simulink model "Red_problema7_lazo_abierto_v2021"  (R2021a)
settings: Solver=ode15s  StartTime=0.0  StopTime=sim_time  RelTol=1e-3
values from neighbouring files (symbols this model uses):
  aE1 = a121_f    (= 50.6984417257)    [inicializar_areas_ej7.m]
  aE2 = a112_f    (= 77.7288481128)    [inicializar_areas_ej7.m]
  aE3 = a222_f    (= 163.424628674)    [inicializar_areas_ej7.m]
  aE4 = a213_f    (= 304.960661681)    [inicializar_areas_ej7.m]
  aEcu1 = aEcu1_f    (= 4.92677788377)    [inicializar_areas_ej7.m]
  aEcu2 = aEcu2_f    (= 18.7854640224)    [inicializar_areas_ej7.m]
  aEhu2 = aEhu2_f    (= 81.1441370104)    [inicializar_areas_ej7.m]
  d1_end = 0    [script_build_tfs.m]    (also in todo_nom_full.m; todo_nom_spar.m)
  d1_in = 0    [script_build_tfs.m]    (also in todo_nom_full.m; todo_nom_spar.m)
  d2_end = 0    [script_build_tfs.m]    (also in todo_nom_full.m; todo_nom_spar.m)
  d2_in = 0    [script_build_tfs.m]    (also in todo_nom_full.m; todo_nom_spar.m)
  d3_end = 0    [script_build_tfs.m]    (also in todo_nom_full.m; todo_nom_spar.m)
  d3_in = 0    [script_build_tfs.m]    (also in todo_nom_full.m; todo_nom_spar.m)
  d4_end = 0    [script_build_tfs.m]    (also in todo_nom_full.m; todo_nom_spar.m)
  d4_in = 0    [script_build_tfs.m]    (also in todo_nom_full.m; todo_nom_spar.m)
  d5_end = 0    [script_build_tfs.m]    (also in todo_nom_full.m; todo_nom_spar.m)
  d5_in = 0    [script_build_tfs.m]    (also in todo_nom_full.m; todo_nom_spar.m)
  d6_end = 0    [script_build_tfs.m]    (also in todo_nom_full.m; todo_nom_spar.m)
  d6_in = 0    [script_build_tfs.m]    (also in todo_nom_full.m; todo_nom_spar.m)
  d7_end = 0    [script_build_tfs.m]    (also in todo_nom_full.m; todo_nom_spar.m)
  d7_in = 0    [script_build_tfs.m]    (also in todo_nom_full.m; todo_nom_spar.m)
  d8_end = 0    [script_build_tfs.m]    (also in todo_nom_full.m; todo_nom_spar.m)
  d8_in = 0    [script_build_tfs.m]    (also in todo_nom_full.m; todo_nom_spar.m)
  fcu2 = 5    [ini_comun.m]    (also in inicializar_areas_ej7.m; script_build_tfs.m; script_ini_ej7.m)
  fhu2 = 15    [ini_comun.m]    (also in inicializar_areas_ej7.m; script_build_tfs.m; script_ini_ej7.m)
  hcu = 1    [ini_comun.m]    (also in script_build_tfs.m; script_ini_ej7.m)
  hhu = 1    [ini_comun.m]    (also in script_build_tfs.m; script_ini_ej7.m)
  s1 = 30    [ini_comun.m]    (also in script_build_tfs.m; script_ini_ej7.m)
  salida_pto_op = [432.98548652 333.041991092 482.910853128 483.037830645]    [D_desc_v1.mat]    (also in D_full_v1.mat = [432.959604691 333.033592475 482.878829311 483.126301479]; D_spar_v1.mat = [433.148784168 333.052277913 483.093095371 482.96198908]; salida_pt_op_desc.mat = [432.94450339 332.966292174 482.988443985 483.057252903]; salida_pt_op_desc_v2021.mat)
  t_step = 2000    [ini_comun.m]    (also in script_build_tfs.m = 300; script_ini_ej7.m = 600; validacion.m = 500)
  Tcuin = 288    [ini_comun.m]    (also in script_build_tfs.m; script_ini_ej7.m)
  Thuin = 523    [ini_comun.m]    (also in script_build_tfs.m; script_ini_ej7.m)
  u10_end = nom_ini(10)    [script_build_tfs.m]    (also in todo_nom_full.m = 0; todo_nom_spar.m = 0; validacion.m)
  u10_in = nom_ini(10)    [script_build_tfs.m]    (also in todo_nom_full.m = 0; todo_nom_spar.m = 0; validacion.m)
  u11_end = nom_ini(11)    [script_build_tfs.m]    (also in todo_nom_full.m = 0; todo_nom_spar.m = 0; validacion.m)
  u11_in = nom_ini(11)    [script_build_tfs.m]    (also in todo_nom_full.m = 0; todo_nom_spar.m = 0; validacion.m)
  u1_end = nom_ini(1)    [script_build_tfs.m]    (also in todo_nom_full.m = nominales_u_full(1); todo_nom_spar.m = nominales_u_spar(1); validacion.m)
  u1_in = nom_ini(1)    [script_build_tfs.m]    (also in todo_nom_full.m = nominales_u_full(1); todo_nom_spar.m = nominales_u_spar(1); validacion.m)
  u2_end = nom_ini(2)    [script_build_tfs.m]    (also in todo_nom_full.m = nominales_u_full(2); todo_nom_spar.m = nominales_u_spar(2); validacion.m)
  u2_in = nom_ini(2)    [script_build_tfs.m]    (also in todo_nom_full.m = nominales_u_full(2); todo_nom_spar.m = nominales_u_spar(2); validacion.m)
  u3_end = nom_ini(3)    [script_build_tfs.m]    (also in todo_nom_full.m = nominales_u_full(3); todo_nom_spar.m = nominales_u_spar(3); validacion.m)
  u3_in = nom_ini(3)    [script_build_tfs.m]    (also in todo_nom_full.m = nominales_u_full(3); todo_nom_spar.m = nominales_u_spar(3); validacion.m)
  u4_end = nom_ini(4)    [script_build_tfs.m]    (also in todo_nom_full.m = nominales_u_full(4); todo_nom_spar.m = nominales_u_spar(4); validacion.m)
  u4_in = nom_ini(4)    [script_build_tfs.m]    (also in todo_nom_full.m = nominales_u_full(4); todo_nom_spar.m = nominales_u_spar(4); validacion.m)
  u5_end = nom_ini(5)    [script_build_tfs.m]    (also in todo_nom_full.m = nominales_u_full(5); todo_nom_spar.m = nominales_u_spar(5); validacion.m)
  u5_in = nom_ini(5)    [script_build_tfs.m]    (also in todo_nom_full.m = nominales_u_full(5); todo_nom_spar.m = nominales_u_spar(5); validacion.m)
  u6_end = nom_ini(6)    [script_build_tfs.m]    (also in todo_nom_full.m = nominales_u_full(6); todo_nom_spar.m = nominales_u_spar(6); validacion.m)
  u6_in = nom_ini(6)    [script_build_tfs.m]    (also in todo_nom_full.m = nominales_u_full(6); todo_nom_spar.m = nominales_u_spar(6); validacion.m)
  u7_end = nom_ini(7)    [script_build_tfs.m]    (also in todo_nom_full.m = nominales_u_full(7); todo_nom_spar.m = nominales_u_spar(7); validacion.m)
  u7_in = nom_ini(7)    [script_build_tfs.m]    (also in todo_nom_full.m = nominales_u_full(7); todo_nom_spar.m = nominales_u_spar(7); validacion.m)
  u8_end = nom_ini(8)    [script_build_tfs.m]    (also in todo_nom_full.m = nominales_u_full(8); todo_nom_spar.m = nominales_u_spar(8); validacion.m)
  u8_in = nom_ini(8)    [script_build_tfs.m]    (also in todo_nom_full.m = nominales_u_full(8); todo_nom_spar.m = nominales_u_spar(8); validacion.m)
  u9_end = nom_ini(9)    [script_build_tfs.m]    (also in todo_nom_full.m = 0; todo_nom_spar.m = 0; validacion.m)
  u9_in = nom_ini(9)    [script_build_tfs.m]    (also in todo_nom_full.m = 0; todo_nom_spar.m = 0; validacion.m)
libraries: simulink x5, cstblocks x1
(part 2 of 2)

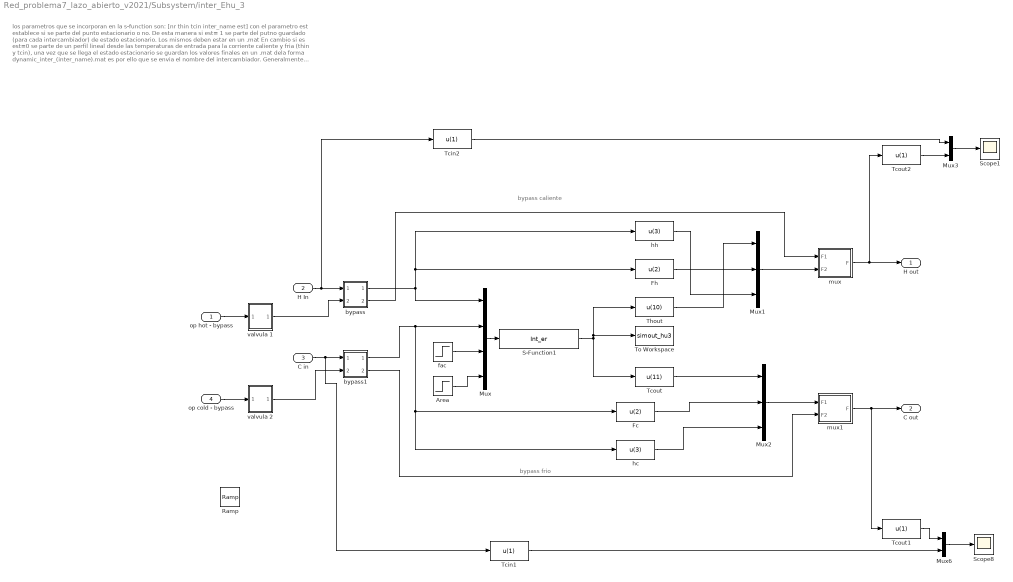
== system Red_problema7_lazo_abierto_v2021/Subsystem/inter_Ehu_3 ==
  note: bypass caliente
  note: bypass frio
  note: los parametros que se incorporan en la s-function son: [nr thin tcin inter_name est]
      | con el parametro est establece si se parte del punto estacionario o no. De esta manera si est= 1 se parte del putno guardado (para cada intercambiador) de estado estacionario. Los mismos deben estar en un .mat
      | En cambio si es est=0 se parte de un perfil lineal  desde las temperaturas de entrada para la corriente caliente y fria (thin y tcin), una vez que se llega el estado estacionario se guardan los valores finales en un .mat
      | dela forma dynamic_inter_(inter_name).mat   es por ello que se envia el nombre del intercambiador.
      | Generalmente para la primera vez que se corre la red se una est=0 para que llegue al estado estacionario y una vez que se alcanzó se vuelve a correr con est= 1 para hacer análisis de control
  "op hot - bypass " : Inport
  H In : Inport  Port=2
  C in : Inport  Port=3
  "op cold - bypass " : Inport  Port=4
  Area : Step  Time=8  Before=aEhu2  After=aEhu2  SampleTime=0
  Fc : Fcn  Expr=u(2)
  Fh : Fcn  Expr=u(2)
  Mux : Mux
  Mux1 : Mux  Inputs=3
  Mux2 : Mux  Inputs=3
  Mux3 : Mux  Inputs=2
  Mux6 : Mux  Inputs=2
  Ramp : simulink/Sources/Ramp  slope=1  start=0  InitialOutput=0
  S-Function1 : S-Function  FunctionName=Int_er  Parameters=10 523 471 03 2  SFunctionDeploymentMode=off  EnableBusSupport=off
  Scope1 : Scope
  Scope8 : Scope
  Tcin1 : Fcn  Expr=u(1)
  Tcin2 : Fcn  Expr=u(1)
  Tcout : Fcn  Expr=u(11)
  Tcout1 : Fcn  Expr=u(1)
  Tcout2 : Fcn  Expr=u(1)
  Thout : Fcn  Expr=u(10)
  To Workspace : ToWorkspace  VariableName=simout_hu3  SampleTime=-1
  bypass : Subsystem
  bypass1 : Subsystem
  fac : Step  After=0  SampleTime=0
  hc : Fcn  Expr=u(3)
  hh : Fcn  Expr=u(3)
  mux : Subsystem
  mux1 : Subsystem
  valvula 1 : Subsystem
  valvula 2 : Subsystem
  H out : Outport  VectorParamsAs1DForOutWhenUnconnected=off
  C out : Outport  Port=2  VectorParamsAs1DForOutWhenUnconnected=off
  wires:
  Tcin2/1 -> Mux3/1
  Tcout2/1 -> Mux3/2
  Mux3/1 -> Scope1/1
  Tcin1/1 -> Mux6/2
  Tcout1/1 -> Mux6/1
  Mux6/1 -> Scope8/1
  bypass1/2(" 2") -> mux1/2(F2)
  bypass1/1(" 1") -> Mux/2, Fc/1, hc/1
  mux1/1("F ") -> C out/1, Tcout1/1
  Mux2/1 -> mux1/1(F1)
  mux/1("F ") -> H out/1, Tcout2/1
  "op cold - bypass "/1 -> valvula 2/1(In1)
  C in/1 -> bypass1/1(1), Tcin1/1
  "op hot - bypass "/1 -> valvula 1/1(In1)
  bypass/2(" 2") -> mux/1(F1)
  Mux1/1 -> mux/2(F2)
  bypass/1(" 1") -> hh/1, Fh/1, Mux/1
  H In/1 -> bypass/1(1), Tcin2/1
  Area/1 -> Mux/4
  hh/1 -> Mux1/3
  hc/1 -> Mux2/3
  fac/1 -> Mux/3
  Mux/1 -> S-Function1/1
  S-Function1/1 -> Tcout/1, To Workspace/1, Thout/1
  Fh/1 -> Mux1/2
  Fc/1 -> Mux2/2
  Thout/1 -> Mux1/1
  Tcout/1 -> Mux2/1
  valvula 1/1(Out1) -> bypass/2(u122)
  valvula 2/1(Out1) -> bypass1/2(u122)

== system Red_problema7_lazo_abierto_v2021/Subsystem/Corriente C1/valvula 3 ==
  In1 : Inport
  Gain : Gain  Gain=s1
  Gain1 : Gain  Gain=s1
  Integrator : Integrator  InitialCondition=[Thuin fhu2 hhu]
  Sum : Sum  Inputs=|+-
  Out1 : Outport  VectorParamsAs1DForOutWhenUnconnected=off
  wires:
  Gain1/1 -> Sum/2
  Integrator/1 -> Out1/1, Gain1/1
  Sum/1 -> Integrator/1
  Gain/1 -> Sum/1
  In1/1 -> Gain/1

== system Red_problema7_lazo_abierto_v2021/Subsystem/Corriente C2/valvula 3 ==
  In1 : Inport
  Gain : Gain  Gain=s1
  Gain1 : Gain  Gain=s1
  Integrator : Integrator  InitialCondition=[Thuin fhu2 hhu]
  Sum : Sum  Inputs=|+-
  Out1 : Outport  VectorParamsAs1DForOutWhenUnconnected=off
  wires:
  Gain1/1 -> Sum/2
  Integrator/1 -> Out1/1, Gain1/1
  Sum/1 -> Integrator/1
  Gain/1 -> Sum/1
  In1/1 -> Gain/1

== system Red_problema7_lazo_abierto_v2021/Subsystem/Corriente H1/valvula 3 ==
  In1 : Inport
  Gain : Gain  Gain=s1
  Gain1 : Gain  Gain=s1
  Integrator : Integrator  InitialCondition=[Thuin fhu2 hhu]
  Sum : Sum  Inputs=|+-
  Out1 : Outport  VectorParamsAs1DForOutWhenUnconnected=off
  wires:
  Gain1/1 -> Sum/2
  Integrator/1 -> Out1/1, Gain1/1
  Sum/1 -> Integrator/1
  Gain/1 -> Sum/1
  In1/1 -> Gain/1

== system Red_problema7_lazo_abierto_v2021/Subsystem/Corriente H2/valvula 3 ==
  In1 : Inport
  Gain : Gain  Gain=s1
  Gain1 : Gain  Gain=s1
  Integrator : Integrator  InitialCondition=[Thuin fhu2 hhu]
  Sum : Sum  Inputs=|+-
  Out1 : Outport  VectorParamsAs1DForOutWhenUnconnected=off
  wires:
  Gain1/1 -> Sum/2
  Integrator/1 -> Out1/1, Gain1/1
  Sum/1 -> Integrator/1
  Gain/1 -> Sum/1
  In1/1 -> Gain/1

== system Red_problema7_lazo_abierto_v2021/Subsystem/Corriente Hu1/valvula 3 ==
  In1 : Inport
  Gain : Gain  Gain=s1
  Gain1 : Gain  Gain=s1
  Integrator : Integrator  InitialCondition=[Tcuin fcu2 hcu]
  Sum : Sum  Inputs=|+-
  Out1 : Outport  VectorParamsAs1DForOutWhenUnconnected=off
  wires:
  Gain1/1 -> Sum/2
  Integrator/1 -> Out1/1, Gain1/1
  Sum/1 -> Integrator/1
  Gain/1 -> Sum/1
  In1/1 -> Gain/1

== system Red_problema7_lazo_abierto_v2021/Subsystem/Corriente Hu2/valvula 3 ==
  In1 : Inport
  Gain : Gain  Gain=s1
  Gain1 : Gain  Gain=s1
  Integrator : Integrator  InitialCondition=[Tcuin fcu2 hcu]
  Sum : Sum  Inputs=|+-
  Out1 : Outport  VectorParamsAs1DForOutWhenUnconnected=off
  wires:
  Gain1/1 -> Sum/2
  Integrator/1 -> Out1/1, Gain1/1
  Sum/1 -> Integrator/1
  Gain/1 -> Sum/1
  In1/1 -> Gain/1

== system Red_problema7_lazo_abierto_v2021/Subsystem/Corriente Hu3/valvula 3 ==
  In1 : Inport
  Gain : Gain  Gain=s1
  Gain1 : Gain  Gain=s1
  Integrator : Integrator  InitialCondition=[Tcuin fcu2 hcu]
  Sum : Sum  Inputs=|+-
  Out1 : Outport  VectorParamsAs1DForOutWhenUnconnected=off
  wires:
  Gain1/1 -> Sum/2
  Integrator/1 -> Out1/1, Gain1/1
  Sum/1 -> Integrator/1
  Gain/1 -> Sum/1
  In1/1 -> Gain/1

== system Red_problema7_lazo_abierto_v2021/Subsystem/inter_E1/bypass ==
  note: la corriete 2 es la corriente del byapass
  note: la corriente 1 es la que se introduce al intercambiador
  1 : Inport
  u122 : Inport  Port=2
  Add : Sum  Inputs=+-
  Mux : Mux  Inputs=3
  Mux1 : Mux  Inputs=3
  Product : Product
  T : Fcn  Expr=u(1)
  f : Fcn  Expr=u(2)
  h : Fcn  Expr=u(3)
  " 1" : Outport  VectorParamsAs1DForOutWhenUnconnected=off
  " 2" : Outport  Port=2  VectorParamsAs1DForOutWhenUnconnected=off
  wires:
  u122/1 -> Product/1
  f/1 -> Add/1, Product/2
  Product/1 -> Mux1/2, Add/2
  1/1 -> T/1, h/1, f/1
  Add/1 -> Mux/2
  h/1 -> Mux1/3, Mux/3
  T/1 -> Mux1/1, Mux/1
  Mux/1 -> " 1"/1
  Mux1/1 -> " 2"/1

== system Red_problema7_lazo_abierto_v2021/Subsystem/inter_E1/bypass1 ==
  note: la corriente 1 es la que se introduce al intercambiador
  note: la corriete 2 es la corriente del byapass
  1 : Inport
  u122 : Inport  Port=2
  Add : Sum  Inputs=+-
  Mux : Mux  Inputs=3
  Mux1 : Mux  Inputs=3
  Product : Product
  T : Fcn  Expr=u(1)
  f : Fcn  Expr=u(2)
  h : Fcn  Expr=u(3)
  " 1" : Outport  VectorParamsAs1DForOutWhenUnconnected=off
  " 2" : Outport  Port=2  VectorParamsAs1DForOutWhenUnconnected=off
  wires:
  Mux1/1 -> " 2"/1
  Mux/1 -> " 1"/1
  T/1 -> Mux/1, Mux1/1
  h/1 -> Mux/3, Mux1/3
  Add/1 -> Mux/2
  1/1 -> f/1, h/1, T/1
  Product/1 -> Add/2, Mux1/2
  f/1 -> Product/2, Add/1
  u122/1 -> Product/1

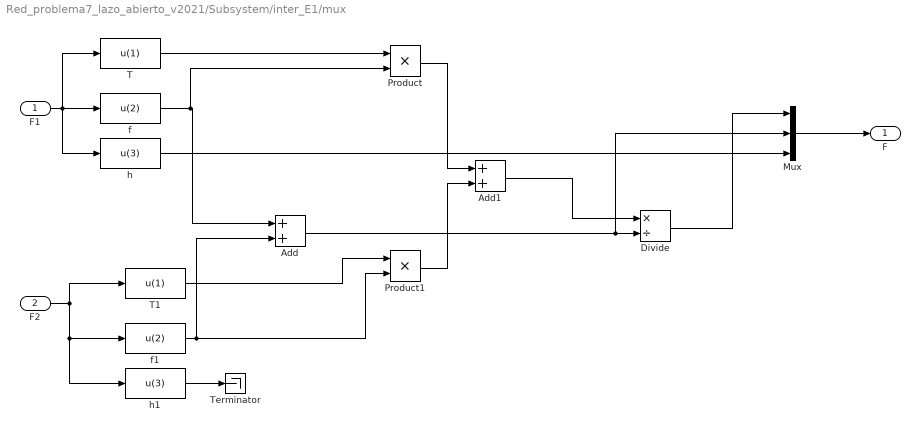
== system Red_problema7_lazo_abierto_v2021/Subsystem/inter_E1/mux ==
  F1 : Inport
  F2 : Inport  Port=2
  Add : Sum
  Add1 : Sum
  Divide : Product  Inputs=*/
  Mux : Mux  Inputs=3
  Product : Product
  Product1 : Product
  T : Fcn  Expr=u(1)
  T1 : Fcn  Expr=u(1)
  Terminator : Terminator
  f : Fcn  Expr=u(2)
  f1 : Fcn  Expr=u(2)
  h : Fcn  Expr=u(3)
  h1 : Fcn  Expr=u(3)
  "F " : Outport  VectorParamsAs1DForOutWhenUnconnected=off
  wires:
  h/1 -> Mux/3
  Divide/1 -> Mux/1
  Add/1 -> Divide/2, Mux/2
  Add1/1 -> Divide/1
  Product1/1 -> Add1/2
  f1/1 -> Product1/2, Add/2
  T1/1 -> Product1/1
  Product/1 -> Add1/1
  T/1 -> Product/1
  F2/1 -> T1/1, f1/1, h1/1
  f/1 -> Add/1, Product/2
  F1/1 -> T/1, h/1, f/1
  Mux/1 -> "F "/1
  h1/1 -> Terminator/1

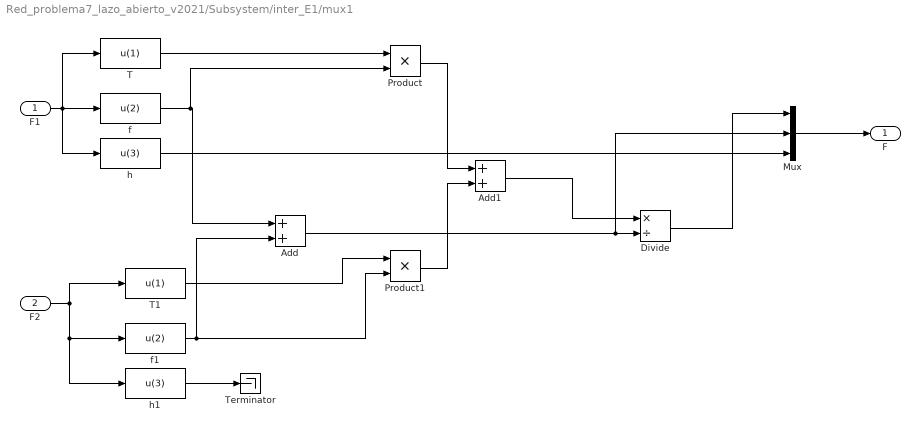
== system Red_problema7_lazo_abierto_v2021/Subsystem/inter_E1/mux1 ==
  F1 : Inport
  F2 : Inport  Port=2
  Add : Sum
  Add1 : Sum
  Divide : Product  Inputs=*/
  Mux : Mux  Inputs=3
  Product : Product
  Product1 : Product
  T : Fcn  Expr=u(1)
  T1 : Fcn  Expr=u(1)
  Terminator : Terminator
  f : Fcn  Expr=u(2)
  f1 : Fcn  Expr=u(2)
  h : Fcn  Expr=u(3)
  h1 : Fcn  Expr=u(3)
  "F " : Outport  VectorParamsAs1DForOutWhenUnconnected=off
  wires:
  Mux/1 -> "F "/1
  F1/1 -> f/1, h/1, T/1
  f/1 -> Product/2, Add/1
  F2/1 -> h1/1, f1/1, T1/1
  T/1 -> Product/1
  Product/1 -> Add1/1
  T1/1 -> Product1/1
  f1/1 -> Add/2, Product1/2
  Product1/1 -> Add1/2
  Add1/1 -> Divide/1
  Add/1 -> Mux/2, Divide/2
  Divide/1 -> Mux/1
  h/1 -> Mux/3
  h1/1 -> Terminator/1

== system Red_problema7_lazo_abierto_v2021/Subsystem/inter_E1/valvula 1 ==
  In1 : Inport
  Gain : Gain  Gain=s1
  Gain1 : Gain  Gain=s1
  Integrator : Integrator
  Sum : Sum  Inputs=|+-
  Out1 : Outport  VectorParamsAs1DForOutWhenUnconnected=off
  wires:
  Gain1/1 -> Sum/2
  Integrator/1 -> Out1/1, Gain1/1
  Sum/1 -> Integrator/1
  Gain/1 -> Sum/1
  In1/1 -> Gain/1

== system Red_problema7_lazo_abierto_v2021/Subsystem/inter_E1/valvula 2 ==
  In1 : Inport
  Gain : Gain  Gain=s1
  Gain1 : Gain  Gain=s1
  Integrator : Integrator
  Sum : Sum  Inputs=|+-
  Out1 : Outport  VectorParamsAs1DForOutWhenUnconnected=off
  wires:
  Gain1/1 -> Sum/2
  Integrator/1 -> Out1/1, Gain1/1
  Sum/1 -> Integrator/1
  Gain/1 -> Sum/1
  In1/1 -> Gain/1

== system Red_problema7_lazo_abierto_v2021/Subsystem/inter_E2/bypass ==
  note: la corriente 1 es la que se introduce al intercambiador
  note: la corriete 2 es la corriente del byapass
  1 : Inport
  u122 : Inport  Port=2
  Add : Sum  Inputs=+-
  Mux : Mux  Inputs=3
  Mux1 : Mux  Inputs=3
  Product : Product
  T : Fcn  Expr=u(1)
  f : Fcn  Expr=u(2)
  h : Fcn  Expr=u(3)
  " 1" : Outport  VectorParamsAs1DForOutWhenUnconnected=off
  " 2" : Outport  Port=2  VectorParamsAs1DForOutWhenUnconnected=off
  wires:
  Mux1/1 -> " 2"/1
  Mux/1 -> " 1"/1
  T/1 -> Mux/1, Mux1/1
  h/1 -> Mux/3, Mux1/3
  Add/1 -> Mux/2
  1/1 -> f/1, h/1, T/1
  Product/1 -> Add/2, Mux1/2
  f/1 -> Product/2, Add/1
  u122/1 -> Product/1

== system Red_problema7_lazo_abierto_v2021/Subsystem/inter_E2/bypass1 ==
  note: la corriete 2 es la corriente del byapass
  note: la corriente 1 es la que se introduce al intercambiador
  1 : Inport
  u122 : Inport  Port=2
  Add : Sum  Inputs=+-
  Mux : Mux  Inputs=3
  Mux1 : Mux  Inputs=3
  Product : Product
  T : Fcn  Expr=u(1)
  f : Fcn  Expr=u(2)
  h : Fcn  Expr=u(3)
  " 1" : Outport  VectorParamsAs1DForOutWhenUnconnected=off
  " 2" : Outport  Port=2  VectorParamsAs1DForOutWhenUnconnected=off
  wires:
  u122/1 -> Product/1
  f/1 -> Add/1, Product/2
  Product/1 -> Mux1/2, Add/2
  1/1 -> T/1, h/1, f/1
  Add/1 -> Mux/2
  h/1 -> Mux1/3, Mux/3
  T/1 -> Mux1/1, Mux/1
  Mux/1 -> " 1"/1
  Mux1/1 -> " 2"/1

== system Red_problema7_lazo_abierto_v2021/Subsystem/inter_E2/mux ==
  F1 : Inport
  F2 : Inport  Port=2
  Add : Sum
  Add1 : Sum
  Divide : Product  Inputs=*/
  Mux : Mux  Inputs=3
  Product : Product
  Product1 : Product
  T : Fcn  Expr=u(1)
  T1 : Fcn  Expr=u(1)
  f : Fcn  Expr=u(2)
  f1 : Fcn  Expr=u(2)
  h : Fcn  Expr=u(3)
  h1 : Fcn  Expr=u(3)
  "F " : Outport  VectorParamsAs1DForOutWhenUnconnected=off
  wires:
  Mux/1 -> "F "/1
  F1/1 -> f/1, h/1, T/1
  f/1 -> Product/2, Add/1
  F2/1 -> h1/1, f1/1, T1/1
  T/1 -> Product/1
  Product/1 -> Add1/1
  T1/1 -> Product1/1
  f1/1 -> Add/2, Product1/2
  Product1/1 -> Add1/2
  Add1/1 -> Divide/1
  Add/1 -> Mux/2, Divide/2
  Divide/1 -> Mux/1
  h/1 -> Mux/3

== system Red_problema7_lazo_abierto_v2021/Subsystem/inter_E2/mux1 ==
  F1 : Inport
  F2 : Inport  Port=2
  Add : Sum
  Add1 : Sum
  Divide : Product  Inputs=*/
  Mux : Mux  Inputs=3
  Product : Product
  Product1 : Product
  T : Fcn  Expr=u(1)
  T1 : Fcn  Expr=u(1)
  f : Fcn  Expr=u(2)
  f1 : Fcn  Expr=u(2)
  h : Fcn  Expr=u(3)
  h1 : Fcn  Expr=u(3)
  "F " : Outport  VectorParamsAs1DForOutWhenUnconnected=off
  wires:
  h/1 -> Mux/3
  Divide/1 -> Mux/1
  Add/1 -> Divide/2, Mux/2
  Add1/1 -> Divide/1
  Product1/1 -> Add1/2
  f1/1 -> Product1/2, Add/2
  T1/1 -> Product1/1
  Product/1 -> Add1/1
  T/1 -> Product/1
  F2/1 -> T1/1, f1/1, h1/1
  f/1 -> Add/1, Product/2
  F1/1 -> T/1, h/1, f/1
  Mux/1 -> "F "/1

== system Red_problema7_lazo_abierto_v2021/Subsystem/inter_E2/valvula 1 ==
  In1 : Inport
  Gain : Gain  Gain=s1
  Gain1 : Gain  Gain=s1
  Integrator : Integrator
  Sum : Sum  Inputs=|+-
  Out1 : Outport  VectorParamsAs1DForOutWhenUnconnected=off
  wires:
  Gain1/1 -> Sum/2
  Integrator/1 -> Out1/1, Gain1/1
  Sum/1 -> Integrator/1
  Gain/1 -> Sum/1
  In1/1 -> Gain/1

== system Red_problema7_lazo_abierto_v2021/Subsystem/inter_E2/valvula 2 ==
  In1 : Inport
  Gain : Gain  Gain=s1
  Gain1 : Gain  Gain=s1
  Integrator : Integrator
  Sum : Sum  Inputs=|+-
  Out1 : Outport  VectorParamsAs1DForOutWhenUnconnected=off
  wires:
  Gain1/1 -> Sum/2
  Integrator/1 -> Out1/1, Gain1/1
  Sum/1 -> Integrator/1
  Gain/1 -> Sum/1
  In1/1 -> Gain/1

== system Red_problema7_lazo_abierto_v2021/Subsystem/inter_E3/bypass ==
  note: la corriente 1 es la que se introduce al intercambiador
  note: la corriete 2 es la corriente del byapass
  1 : Inport
  u122 : Inport  Port=2
  Add : Sum  Inputs=+-
  Mux : Mux  Inputs=3
  Mux1 : Mux  Inputs=3
  Product : Product
  T : Fcn  Expr=u(1)
  f : Fcn  Expr=u(2)
  h : Fcn  Expr=u(3)
  " 1" : Outport  VectorParamsAs1DForOutWhenUnconnected=off
  " 2" : Outport  Port=2  VectorParamsAs1DForOutWhenUnconnected=off
  wires:
  Mux1/1 -> " 2"/1
  Mux/1 -> " 1"/1
  T/1 -> Mux/1, Mux1/1
  h/1 -> Mux/3, Mux1/3
  Add/1 -> Mux/2
  1/1 -> f/1, h/1, T/1
  Product/1 -> Add/2, Mux1/2
  f/1 -> Product/2, Add/1
  u122/1 -> Product/1

== system Red_problema7_lazo_abierto_v2021/Subsystem/inter_E3/bypass1 ==
  note: la corriete 2 es la corriente del byapass
  note: la corriente 1 es la que se introduce al intercambiador
  1 : Inport
  u122 : Inport  Port=2
  Add : Sum  Inputs=+-
  Mux : Mux  Inputs=3
  Mux1 : Mux  Inputs=3
  Product : Product
  T : Fcn  Expr=u(1)
  f : Fcn  Expr=u(2)
  h : Fcn  Expr=u(3)
  " 1" : Outport  VectorParamsAs1DForOutWhenUnconnected=off
  " 2" : Outport  Port=2  VectorParamsAs1DForOutWhenUnconnected=off
  wires:
  u122/1 -> Product/1
  f/1 -> Add/1, Product/2
  Product/1 -> Mux1/2, Add/2
  1/1 -> T/1, h/1, f/1
  Add/1 -> Mux/2
  h/1 -> Mux1/3, Mux/3
  T/1 -> Mux1/1, Mux/1
  Mux/1 -> " 1"/1
  Mux1/1 -> " 2"/1

== system Red_problema7_lazo_abierto_v2021/Subsystem/inter_E3/mux ==
  F1 : Inport
  F2 : Inport  Port=2
  Add : Sum
  Add1 : Sum
  Divide : Product  Inputs=*/
  Mux : Mux  Inputs=3
  Product : Product
  Product1 : Product
  T : Fcn  Expr=u(1)
  T1 : Fcn  Expr=u(1)
  f : Fcn  Expr=u(2)
  f1 : Fcn  Expr=u(2)
  h : Fcn  Expr=u(3)
  h1 : Fcn  Expr=u(3)
  "F " : Outport  VectorParamsAs1DForOutWhenUnconnected=off
  wires:
  Mux/1 -> "F "/1
  F1/1 -> f/1, h/1, T/1
  f/1 -> Product/2, Add/1
  F2/1 -> h1/1, f1/1, T1/1
  T/1 -> Product/1
  Product/1 -> Add1/1
  T1/1 -> Product1/1
  f1/1 -> Add/2, Product1/2
  Product1/1 -> Add1/2
  Add1/1 -> Divide/1
  Add/1 -> Mux/2, Divide/2
  Divide/1 -> Mux/1
  h/1 -> Mux/3

== system Red_problema7_lazo_abierto_v2021/Subsystem/inter_E3/mux1 ==
  F1 : Inport
  F2 : Inport  Port=2
  Add : Sum
  Add1 : Sum
  Divide : Product  Inputs=*/
  Mux : Mux  Inputs=3
  Product : Product
  Product1 : Product
  T : Fcn  Expr=u(1)
  T1 : Fcn  Expr=u(1)
  f : Fcn  Expr=u(2)
  f1 : Fcn  Expr=u(2)
  h : Fcn  Expr=u(3)
  h1 : Fcn  Expr=u(3)
  "F " : Outport  VectorParamsAs1DForOutWhenUnconnected=off
  wires:
  h/1 -> Mux/3
  Divide/1 -> Mux/1
  Add/1 -> Divide/2, Mux/2
  Add1/1 -> Divide/1
  Product1/1 -> Add1/2
  f1/1 -> Product1/2, Add/2
  T1/1 -> Product1/1
  Product/1 -> Add1/1
  T/1 -> Product/1
  F2/1 -> T1/1, f1/1, h1/1
  f/1 -> Add/1, Product/2
  F1/1 -> T/1, h/1, f/1
  Mux/1 -> "F "/1

== system Red_problema7_lazo_abierto_v2021/Subsystem/inter_E3/valvula 1 ==
  In1 : Inport
  Gain : Gain  Gain=s1
  Gain1 : Gain  Gain=s1
  Integrator : Integrator
  Sum : Sum  Inputs=|+-
  Out1 : Outport  VectorParamsAs1DForOutWhenUnconnected=off
  wires:
  Gain1/1 -> Sum/2
  Integrator/1 -> Out1/1, Gain1/1
  Sum/1 -> Integrator/1
  Gain/1 -> Sum/1
  In1/1 -> Gain/1

== system Red_problema7_lazo_abierto_v2021/Subsystem/inter_E3/valvula 2 ==
  In1 : Inport
  Gain : Gain  Gain=s1
  Gain1 : Gain  Gain=s1
  Integrator : Integrator
  Sum : Sum  Inputs=|+-
  Out1 : Outport  VectorParamsAs1DForOutWhenUnconnected=off
  wires:
  Gain1/1 -> Sum/2
  Integrator/1 -> Out1/1, Gain1/1
  Sum/1 -> Integrator/1
  Gain/1 -> Sum/1
  In1/1 -> Gain/1

== system Red_problema7_lazo_abierto_v2021/Subsystem/inter_E4/bypass ==
  note: la corriente 1 es la que se introduce al intercambiador
  note: la corriete 2 es la corriente del byapass
  1 : Inport
  u122 : Inport  Port=2
  Add : Sum  Inputs=+-
  Mux : Mux  Inputs=3
  Mux1 : Mux  Inputs=3
  Product : Product
  T : Fcn  Expr=u(1)
  f : Fcn  Expr=u(2)
  h : Fcn  Expr=u(3)
  " 1" : Outport  VectorParamsAs1DForOutWhenUnconnected=off
  " 2" : Outport  Port=2  VectorParamsAs1DForOutWhenUnconnected=off
  wires:
  Mux1/1 -> " 2"/1
  Mux/1 -> " 1"/1
  T/1 -> Mux/1, Mux1/1
  h/1 -> Mux/3, Mux1/3
  Add/1 -> Mux/2
  1/1 -> f/1, h/1, T/1
  Product/1 -> Add/2, Mux1/2
  f/1 -> Product/2, Add/1
  u122/1 -> Product/1

== system Red_problema7_lazo_abierto_v2021/Subsystem/inter_E4/bypass1 ==
  note: la corriete 2 es la corriente del byapass
  note: la corriente 1 es la que se introduce al intercambiador
  1 : Inport
  u122 : Inport  Port=2
  Add : Sum  Inputs=+-
  Mux : Mux  Inputs=3
  Mux1 : Mux  Inputs=3
  Product : Product
  T : Fcn  Expr=u(1)
  f : Fcn  Expr=u(2)
  h : Fcn  Expr=u(3)
  " 1" : Outport  VectorParamsAs1DForOutWhenUnconnected=off
  " 2" : Outport  Port=2  VectorParamsAs1DForOutWhenUnconnected=off
  wires:
  u122/1 -> Product/1
  f/1 -> Add/1, Product/2
  Product/1 -> Mux1/2, Add/2
  1/1 -> T/1, h/1, f/1
  Add/1 -> Mux/2
  h/1 -> Mux1/3, Mux/3
  T/1 -> Mux1/1, Mux/1
  Mux/1 -> " 1"/1
  Mux1/1 -> " 2"/1

== system Red_problema7_lazo_abierto_v2021/Subsystem/inter_E4/mux ==
  F1 : Inport
  F2 : Inport  Port=2
  Add : Sum
  Add1 : Sum
  Divide : Product  Inputs=*/
  Mux : Mux  Inputs=3
  Product : Product
  Product1 : Product
  T : Fcn  Expr=u(1)
  T1 : Fcn  Expr=u(1)
  f : Fcn  Expr=u(2)
  f1 : Fcn  Expr=u(2)
  h : Fcn  Expr=u(3)
  h1 : Fcn  Expr=u(3)
  "F " : Outport  VectorParamsAs1DForOutWhenUnconnected=off
  wires:
  Mux/1 -> "F "/1
  F1/1 -> f/1, h/1, T/1
  f/1 -> Product/2, Add/1
  F2/1 -> h1/1, f1/1, T1/1
  T/1 -> Product/1
  Product/1 -> Add1/1
  T1/1 -> Product1/1
  f1/1 -> Add/2, Product1/2
  Product1/1 -> Add1/2
  Add1/1 -> Divide/1
  Add/1 -> Mux/2, Divide/2
  Divide/1 -> Mux/1
  h/1 -> Mux/3

== system Red_problema7_lazo_abierto_v2021/Subsystem/inter_E4/mux1 ==
  F1 : Inport
  F2 : Inport  Port=2
  Add : Sum
  Add1 : Sum
  Divide : Product  Inputs=*/
  Mux : Mux  Inputs=3
  Product : Product
  Product1 : Product
  T : Fcn  Expr=u(1)
  T1 : Fcn  Expr=u(1)
  f : Fcn  Expr=u(2)
  f1 : Fcn  Expr=u(2)
  h : Fcn  Expr=u(3)
  h1 : Fcn  Expr=u(3)
  "F " : Outport  VectorParamsAs1DForOutWhenUnconnected=off
  wires:
  h/1 -> Mux/3
  Divide/1 -> Mux/1
  Add/1 -> Divide/2, Mux/2
  Add1/1 -> Divide/1
  Product1/1 -> Add1/2
  f1/1 -> Product1/2, Add/2
  T1/1 -> Product1/1
  Product/1 -> Add1/1
  T/1 -> Product/1
  F2/1 -> T1/1, f1/1, h1/1
  f/1 -> Add/1, Product/2
  F1/1 -> T/1, h/1, f/1
  Mux/1 -> "F "/1

== system Red_problema7_lazo_abierto_v2021/Subsystem/inter_E4/valvula 1 ==
  In1 : Inport
  Gain : Gain  Gain=s1
  Gain1 : Gain  Gain=s1
  Integrator : Integrator
  Sum : Sum  Inputs=|+-
  Out1 : Outport  VectorParamsAs1DForOutWhenUnconnected=off
  wires:
  Gain1/1 -> Sum/2
  Integrator/1 -> Out1/1, Gain1/1
  Sum/1 -> Integrator/1
  Gain/1 -> Sum/1
  In1/1 -> Gain/1

== system Red_problema7_lazo_abierto_v2021/Subsystem/inter_E4/valvula 2 ==
  In1 : Inport
  Gain : Gain  Gain=s1
  Gain1 : Gain  Gain=s1
  Integrator : Integrator
  Sum : Sum  Inputs=|+-
  Out1 : Outport  VectorParamsAs1DForOutWhenUnconnected=off
  wires:
  Gain1/1 -> Sum/2
  Integrator/1 -> Out1/1, Gain1/1
  Sum/1 -> Integrator/1
  Gain/1 -> Sum/1
  In1/1 -> Gain/1

== system Red_problema7_lazo_abierto_v2021/Subsystem/inter_Ecu_1/bypass ==
  note: la corriente 1 es la que se introduce al intercambiador
  note: la corriete 2 es la corriente del byapass
  1 : Inport
  u122 : Inport  Port=2
  Add : Sum  Inputs=+-
  Mux : Mux  Inputs=3
  Mux1 : Mux  Inputs=3
  Product : Product
  T : Fcn  Expr=u(1)
  f : Fcn  Expr=u(2)
  h : Fcn  Expr=u(3)
  " 1" : Outport  VectorParamsAs1DForOutWhenUnconnected=off
  " 2" : Outport  Port=2  VectorParamsAs1DForOutWhenUnconnected=off
  wires:
  Mux1/1 -> " 2"/1
  Mux/1 -> " 1"/1
  T/1 -> Mux/1, Mux1/1
  h/1 -> Mux/3, Mux1/3
  Add/1 -> Mux/2
  1/1 -> f/1, h/1, T/1
  Product/1 -> Add/2, Mux1/2
  f/1 -> Product/2, Add/1
  u122/1 -> Product/1

== system Red_problema7_lazo_abierto_v2021/Subsystem/inter_Ecu_1/bypass1 ==
  note: la corriete 2 es la corriente del byapass
  note: la corriente 1 es la que se introduce al intercambiador
  1 : Inport
  u122 : Inport  Port=2
  Add : Sum  Inputs=+-
  Mux : Mux  Inputs=3
  Mux1 : Mux  Inputs=3
  Product : Product
  T : Fcn  Expr=u(1)
  f : Fcn  Expr=u(2)
  h : Fcn  Expr=u(3)
  " 1" : Outport  VectorParamsAs1DForOutWhenUnconnected=off
  " 2" : Outport  Port=2  VectorParamsAs1DForOutWhenUnconnected=off
  wires:
  u122/1 -> Product/1
  f/1 -> Add/1, Product/2
  Product/1 -> Mux1/2, Add/2
  1/1 -> T/1, h/1, f/1
  Add/1 -> Mux/2
  h/1 -> Mux1/3, Mux/3
  T/1 -> Mux1/1, Mux/1
  Mux/1 -> " 1"/1
  Mux1/1 -> " 2"/1

== system Red_problema7_lazo_abierto_v2021/Subsystem/inter_Ecu_1/mux ==
  F1 : Inport
  F2 : Inport  Port=2
  Add : Sum
  Add1 : Sum
  Divide : Product  Inputs=*/
  Mux : Mux  Inputs=3
  Product : Product
  Product1 : Product
  T : Fcn  Expr=u(1)
  T1 : Fcn  Expr=u(1)
  f : Fcn  Expr=u(2)
  f1 : Fcn  Expr=u(2)
  h : Fcn  Expr=u(3)
  h1 : Fcn  Expr=u(3)
  "F " : Outport  VectorParamsAs1DForOutWhenUnconnected=off
  wires:
  Mux/1 -> "F "/1
  F1/1 -> f/1, h/1, T/1
  f/1 -> Product/2, Add/1
  F2/1 -> h1/1, f1/1, T1/1
  T/1 -> Product/1
  Product/1 -> Add1/1
  T1/1 -> Product1/1
  f1/1 -> Add/2, Product1/2
  Product1/1 -> Add1/2
  Add1/1 -> Divide/1
  Add/1 -> Mux/2, Divide/2
  Divide/1 -> Mux/1
  h/1 -> Mux/3

== system Red_problema7_lazo_abierto_v2021/Subsystem/inter_Ecu_1/mux1 ==
  F1 : Inport
  F2 : Inport  Port=2
  Add : Sum
  Add1 : Sum
  Divide : Product  Inputs=*/
  Mux : Mux  Inputs=3
  Product : Product
  Product1 : Product
  T : Fcn  Expr=u(1)
  T1 : Fcn  Expr=u(1)
  f : Fcn  Expr=u(2)
  f1 : Fcn  Expr=u(2)
  h : Fcn  Expr=u(3)
  h1 : Fcn  Expr=u(3)
  "F " : Outport  VectorParamsAs1DForOutWhenUnconnected=off
  wires:
  h/1 -> Mux/3
  Divide/1 -> Mux/1
  Add/1 -> Divide/2, Mux/2
  Add1/1 -> Divide/1
  Product1/1 -> Add1/2
  f1/1 -> Product1/2, Add/2
  T1/1 -> Product1/1
  Product/1 -> Add1/1
  T/1 -> Product/1
  F2/1 -> T1/1, f1/1, h1/1
  f/1 -> Add/1, Product/2
  F1/1 -> T/1, h/1, f/1
  Mux/1 -> "F "/1

== system Red_problema7_lazo_abierto_v2021/Subsystem/inter_Ecu_1/valvula 1 ==
  In1 : Inport
  Gain : Gain  Gain=s1
  Gain1 : Gain  Gain=s1
  Integrator : Integrator
  Sum : Sum  Inputs=|+-
  Out1 : Outport  VectorParamsAs1DForOutWhenUnconnected=off
  wires:
  Gain1/1 -> Sum/2
  Integrator/1 -> Out1/1, Gain1/1
  Sum/1 -> Integrator/1
  Gain/1 -> Sum/1
  In1/1 -> Gain/1

== system Red_problema7_lazo_abierto_v2021/Subsystem/inter_Ecu_1/valvula 2 ==
  In1 : Inport
  Gain : Gain  Gain=s1
  Gain1 : Gain  Gain=s1
  Integrator : Integrator
  Sum : Sum  Inputs=|+-
  Out1 : Outport  VectorParamsAs1DForOutWhenUnconnected=off
  wires:
  Gain1/1 -> Sum/2
  Integrator/1 -> Out1/1, Gain1/1
  Sum/1 -> Integrator/1
  Gain/1 -> Sum/1
  In1/1 -> Gain/1

== system Red_problema7_lazo_abierto_v2021/Subsystem/inter_Ecu_2/bypass ==
  note: la corriente 1 es la que se introduce al intercambiador
  note: la corriete 2 es la corriente del byapass
  1 : Inport
  u122 : Inport  Port=2
  Add : Sum  Inputs=+-
  Mux : Mux  Inputs=3
  Mux1 : Mux  Inputs=3
  Product : Product
  T : Fcn  Expr=u(1)
  f : Fcn  Expr=u(2)
  h : Fcn  Expr=u(3)
  " 1" : Outport  VectorParamsAs1DForOutWhenUnconnected=off
  " 2" : Outport  Port=2  VectorParamsAs1DForOutWhenUnconnected=off
  wires:
  Mux1/1 -> " 2"/1
  Mux/1 -> " 1"/1
  T/1 -> Mux/1, Mux1/1
  h/1 -> Mux/3, Mux1/3
  Add/1 -> Mux/2
  1/1 -> f/1, h/1, T/1
  Product/1 -> Add/2, Mux1/2
  f/1 -> Product/2, Add/1
  u122/1 -> Product/1

== system Red_problema7_lazo_abierto_v2021/Subsystem/inter_Ecu_2/bypass1 ==
  note: la corriete 2 es la corriente del byapass
  note: la corriente 1 es la que se introduce al intercambiador
  1 : Inport
  u122 : Inport  Port=2
  Add : Sum  Inputs=+-
  Mux : Mux  Inputs=3
  Mux1 : Mux  Inputs=3
  Product : Product
  T : Fcn  Expr=u(1)
  f : Fcn  Expr=u(2)
  h : Fcn  Expr=u(3)
  " 1" : Outport  VectorParamsAs1DForOutWhenUnconnected=off
  " 2" : Outport  Port=2  VectorParamsAs1DForOutWhenUnconnected=off
  wires:
  u122/1 -> Product/1
  f/1 -> Add/1, Product/2
  Product/1 -> Mux1/2, Add/2
  1/1 -> T/1, h/1, f/1
  Add/1 -> Mux/2
  h/1 -> Mux1/3, Mux/3
  T/1 -> Mux1/1, Mux/1
  Mux/1 -> " 1"/1
  Mux1/1 -> " 2"/1

== system Red_problema7_lazo_abierto_v2021/Subsystem/inter_Ecu_2/mux ==
  F1 : Inport
  F2 : Inport  Port=2
  Add : Sum
  Add1 : Sum
  Divide : Product  Inputs=*/
  Mux : Mux  Inputs=3
  Product : Product
  Product1 : Product
  T : Fcn  Expr=u(1)
  T1 : Fcn  Expr=u(1)
  f : Fcn  Expr=u(2)
  f1 : Fcn  Expr=u(2)
  h : Fcn  Expr=u(3)
  h1 : Fcn  Expr=u(3)
  "F " : Outport  VectorParamsAs1DForOutWhenUnconnected=off
  wires:
  Mux/1 -> "F "/1
  F1/1 -> f/1, h/1, T/1
  f/1 -> Product/2, Add/1
  F2/1 -> h1/1, f1/1, T1/1
  T/1 -> Product/1
  Product/1 -> Add1/1
  T1/1 -> Product1/1
  f1/1 -> Add/2, Product1/2
  Product1/1 -> Add1/2
  Add1/1 -> Divide/1
  Add/1 -> Mux/2, Divide/2
  Divide/1 -> Mux/1
  h/1 -> Mux/3

== system Red_problema7_lazo_abierto_v2021/Subsystem/inter_Ecu_2/mux1 ==
  F1 : Inport
  F2 : Inport  Port=2
  Add : Sum
  Add1 : Sum
  Divide : Product  Inputs=*/
  Mux : Mux  Inputs=3
  Product : Product
  Product1 : Product
  T : Fcn  Expr=u(1)
  T1 : Fcn  Expr=u(1)
  f : Fcn  Expr=u(2)
  f1 : Fcn  Expr=u(2)
  h : Fcn  Expr=u(3)
  h1 : Fcn  Expr=u(3)
  "F " : Outport  VectorParamsAs1DForOutWhenUnconnected=off
  wires:
  h/1 -> Mux/3
  Divide/1 -> Mux/1
  Add/1 -> Divide/2, Mux/2
  Add1/1 -> Divide/1
  Product1/1 -> Add1/2
  f1/1 -> Product1/2, Add/2
  T1/1 -> Product1/1
  Product/1 -> Add1/1
  T/1 -> Product/1
  F2/1 -> T1/1, f1/1, h1/1
  f/1 -> Add/1, Product/2
  F1/1 -> T/1, h/1, f/1
  Mux/1 -> "F "/1

== system Red_problema7_lazo_abierto_v2021/Subsystem/inter_Ecu_2/valvula 1 ==
  In1 : Inport
  Gain : Gain  Gain=s1
  Gain1 : Gain  Gain=s1
  Integrator : Integrator
  Sum : Sum  Inputs=|+-
  Out1 : Outport  VectorParamsAs1DForOutWhenUnconnected=off
  wires:
  Gain1/1 -> Sum/2
  Integrator/1 -> Out1/1, Gain1/1
  Sum/1 -> Integrator/1
  Gain/1 -> Sum/1
  In1/1 -> Gain/1

== system Red_problema7_lazo_abierto_v2021/Subsystem/inter_Ecu_2/valvula 2 ==
  In1 : Inport
  Gain : Gain  Gain=s1
  Gain1 : Gain  Gain=s1
  Integrator : Integrator
  Sum : Sum  Inputs=|+-
  Out1 : Outport  VectorParamsAs1DForOutWhenUnconnected=off
  wires:
  Gain1/1 -> Sum/2
  Integrator/1 -> Out1/1, Gain1/1
  Sum/1 -> Integrator/1
  Gain/1 -> Sum/1
  In1/1 -> Gain/1

== system Red_problema7_lazo_abierto_v2021/Subsystem/inter_Ehu_3/bypass ==
  note: la corriente 1 es la que se introduce al intercambiador
  note: la corriete 2 es la corriente del byapass
  1 : Inport
  u122 : Inport  Port=2
  Add : Sum  Inputs=+-
  Mux : Mux  Inputs=3
  Mux1 : Mux  Inputs=3
  Product : Product
  T : Fcn  Expr=u(1)
  f : Fcn  Expr=u(2)
  h : Fcn  Expr=u(3)
  " 1" : Outport  VectorParamsAs1DForOutWhenUnconnected=off
  " 2" : Outport  Port=2  VectorParamsAs1DForOutWhenUnconnected=off
  wires:
  Mux1/1 -> " 2"/1
  Mux/1 -> " 1"/1
  T/1 -> Mux/1, Mux1/1
  h/1 -> Mux/3, Mux1/3
  Add/1 -> Mux/2
  1/1 -> f/1, h/1, T/1
  Product/1 -> Add/2, Mux1/2
  f/1 -> Product/2, Add/1
  u122/1 -> Product/1

== system Red_problema7_lazo_abierto_v2021/Subsystem/inter_Ehu_3/bypass1 ==
  note: la corriete 2 es la corriente del byapass
  note: la corriente 1 es la que se introduce al intercambiador
  1 : Inport
  u122 : Inport  Port=2
  Add : Sum  Inputs=+-
  Mux : Mux  Inputs=3
  Mux1 : Mux  Inputs=3
  Product : Product
  T : Fcn  Expr=u(1)
  f : Fcn  Expr=u(2)
  h : Fcn  Expr=u(3)
  " 1" : Outport  VectorParamsAs1DForOutWhenUnconnected=off
  " 2" : Outport  Port=2  VectorParamsAs1DForOutWhenUnconnected=off
  wires:
  u122/1 -> Product/1
  f/1 -> Add/1, Product/2
  Product/1 -> Mux1/2, Add/2
  1/1 -> T/1, h/1, f/1
  Add/1 -> Mux/2
  h/1 -> Mux1/3, Mux/3
  T/1 -> Mux1/1, Mux/1
  Mux/1 -> " 1"/1
  Mux1/1 -> " 2"/1

== system Red_problema7_lazo_abierto_v2021/Subsystem/inter_Ehu_3/mux ==
  F1 : Inport
  F2 : Inport  Port=2
  Add : Sum
  Add1 : Sum
  Divide : Product  Inputs=*/
  Mux : Mux  Inputs=3
  Product : Product
  Product1 : Product
  T : Fcn  Expr=u(1)
  T1 : Fcn  Expr=u(1)
  f : Fcn  Expr=u(2)
  f1 : Fcn  Expr=u(2)
  h : Fcn  Expr=u(3)
  h1 : Fcn  Expr=u(3)
  "F " : Outport  VectorParamsAs1DForOutWhenUnconnected=off
  wires:
  Mux/1 -> "F "/1
  F1/1 -> f/1, h/1, T/1
  f/1 -> Product/2, Add/1
  F2/1 -> h1/1, f1/1, T1/1
  T/1 -> Product/1
  Product/1 -> Add1/1
  T1/1 -> Product1/1
  f1/1 -> Add/2, Product1/2
  Product1/1 -> Add1/2
  Add1/1 -> Divide/1
  Add/1 -> Mux/2, Divide/2
  Divide/1 -> Mux/1
  h/1 -> Mux/3

== system Red_problema7_lazo_abierto_v2021/Subsystem/inter_Ehu_3/mux1 ==
  F1 : Inport
  F2 : Inport  Port=2
  Add : Sum
  Add1 : Sum
  Divide : Product  Inputs=*/
  Mux : Mux  Inputs=3
  Product : Product
  Product1 : Product
  T : Fcn  Expr=u(1)
  T1 : Fcn  Expr=u(1)
  f : Fcn  Expr=u(2)
  f1 : Fcn  Expr=u(2)
  h : Fcn  Expr=u(3)
  h1 : Fcn  Expr=u(3)
  "F " : Outport  VectorParamsAs1DForOutWhenUnconnected=off
  wires:
  h/1 -> Mux/3
  Divide/1 -> Mux/1
  Add/1 -> Divide/2, Mux/2
  Add1/1 -> Divide/1
  Product1/1 -> Add1/2
  f1/1 -> Product1/2, Add/2
  T1/1 -> Product1/1
  Product/1 -> Add1/1
  T/1 -> Product/1
  F2/1 -> T1/1, f1/1, h1/1
  f/1 -> Add/1, Product/2
  F1/1 -> T/1, h/1, f/1
  Mux/1 -> "F "/1

== system Red_problema7_lazo_abierto_v2021/Subsystem/inter_Ehu_3/valvula 1 ==
  In1 : Inport
  Gain : Gain  Gain=s1
  Gain1 : Gain  Gain=s1
  Integrator : Integrator
  Sum : Sum  Inputs=|+-
  Out1 : Outport  VectorParamsAs1DForOutWhenUnconnected=off
  wires:
  Gain1/1 -> Sum/2
  Integrator/1 -> Out1/1, Gain1/1
  Sum/1 -> Integrator/1
  Gain/1 -> Sum/1
  In1/1 -> Gain/1

== system Red_problema7_lazo_abierto_v2021/Subsystem/inter_Ehu_3/valvula 2 ==
  In1 : Inport
  Gain : Gain  Gain=s1
  Gain1 : Gain  Gain=s1
  Integrator : Integrator
  Sum : Sum  Inputs=|+-
  Out1 : Outport  VectorParamsAs1DForOutWhenUnconnected=off
  wires:
  Gain1/1 -> Sum/2
  Integrator/1 -> Out1/1, Gain1/1
  Sum/1 -> Integrator/1
  Gain/1 -> Sum/1
  In1/1 -> Gain/1
